simulink model "TwoLinkCartesianNN"  (Simulink 7.6)
settings: Solver=ode45  StartTime=0.0  StopTime=10.0  RelTol=1e-3
libraries: neural x148, roblocks x3, simulink x1
(part 5 of 5)

== matlab function Embedded MATLAB Function2 ==
  data: q input double; fe output double; X input double
function fe = fcn(q,X)
k = 150000;
z = q(1);
x = q(2);
if  (z>.5 && z<.6) || x<.5
    fe = [0;0];
else
     fe1 = 0;
     fe2 = k*(x-X(2));
     fe = [fe1;fe2];
end

== matlab function Embedded MATLAB Function3 ==
  data: tr output double; c input double
function tr = fcn(c)

% if c < 8
% tr = [.55 ; 0];
% else
%     tr = [.55 ; 1];
% end
% 
tr = [.6;.6];

== matlab function Embedded MATLAB Function ==
  data: f input double; qdd output double
function qdd= fcn(f)
m1 = 1;
m2 = 1;
g = 9.8;
M = [m1+m2 , 0; 0,m2];
G = [g*(m1+m2);0];
qdd = inv(M)*(f-G) ;

== matlab function Embedded MATLAB Function1 ==
  data: v input double; f output double
function f = fcn(v)

m1 = 1;
m2 = 1;
g = 9.8;
M = [m1+m2 , 0; 0,m2];
G = [g*(m1+m2);0];
f = G+M*v;
